simulink model "integrator_12B"  (R2022b)
settings: Solver=VariableStepAuto  StartTime=0.0  StopTime=20  RelTol=1e-3
values from neighbouring files (symbols this model uses):
  BL = -10    [SettingTUI.m]
  TL = 10    [SettingTUI.m]
undefined symbols (not defined in the file or in its folder): Hecate_Amp, Hecate_Freq
libraries: simulink x1
settings Model: LastModifiedBy=fedformi_new
settings DataIOCC: SaveFormat=Array  TimeSaveName=tOut  OutputSaveName=yOut
settings OptimizationCC: BlockReduction=off  BooleanDataType=off
settings DebuggingCC: SaveWithParameterizedLinksMsg=none  UnderspecifiedInitializationDetection=Classic  MergeDetectMultiDrivingBlocksExec=none  SignalResolutionControl=TryResolveAllWithWarning
settings HardwareCC: TargetUnknown=on
settings ModelReferenceCC: EnableRefExpFcnMdlSchedulingChecks=on  PropagateSignalLabelsOutOfModel=off

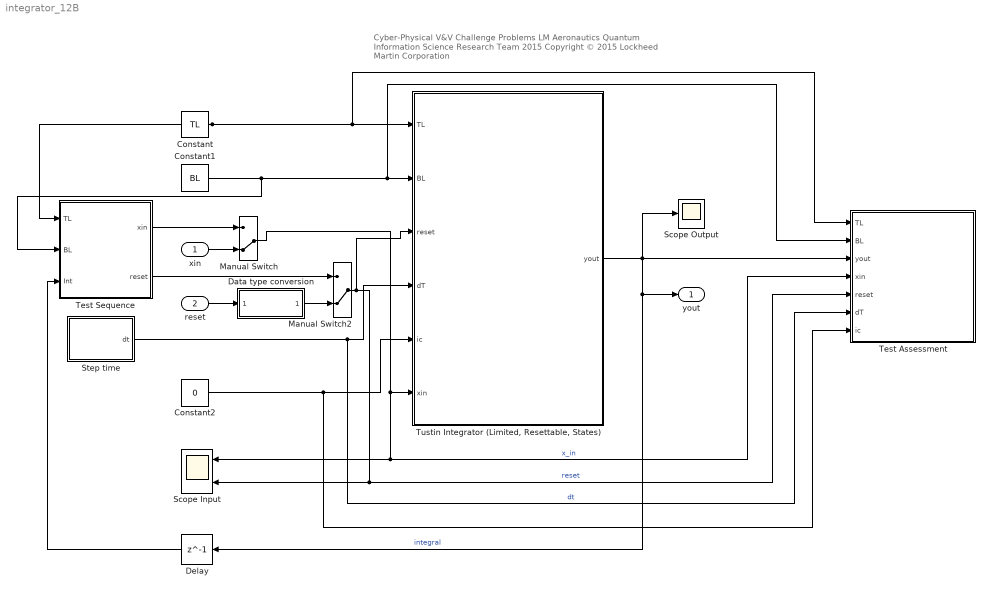
== system integrator_12B ==
  note: Cyber-Physical V&V Challenge Problems
      | LM Aeronautics Quantum Information Science Research Team 2015
      | Copyright © 2015 Lockheed Martin Corporation
  xin : Inport  OutDataTypeStr=double
  reset : Inport  Port=2
  Constant : Constant  Value=TL
  Constant1 : Constant  Value=BL
  Constant2 : Constant  Value=0
  Data type conversion : Subsystem
  Delay : Delay  DelayLength=1  InitialCondition=0
  Manual Switch : ManualSwitch  CurrentSetting=0
  Manual Switch2 : ManualSwitch  CurrentSetting=0
  Scope Input : Scope  NumInputPorts=2
  Scope Output : Scope
  Step time : Subsystem
  Test Assessment : Test Sequence  TreatAsAtomicUnit=on
  Test Sequence : Test Sequence  TreatAsAtomicUnit=on
  "Tustin Integrator (Limited, Resettable, States)" : Subsystem
  yout : Outport
  wires:
  "Tustin Integrator (Limited, Resettable, States)"/1(yout) -> Delay/1, yout/1, Scope Output/1, Test Assessment/3(yout)  "integral"
  Manual Switch/1 -> "Tustin Integrator (Limited, Resettable, States)"/6(xin), Scope Input/1, Test Assessment/4(xin)  "x_in"
  Test Sequence/1(xin) -> Manual Switch/1
  xin/1 -> Manual Switch/2
  Test Sequence/2(reset) -> Manual Switch2/1
  Constant/1 -> "Tustin Integrator (Limited, Resettable, States)"/1(TL), Test Assessment/1(TL), Test Sequence/1(TL)
  Constant1/1 -> Test Sequence/2(BL), "Tustin Integrator (Limited, Resettable, States)"/2(BL), Test Assessment/2(BL)
  Step time/1(dt) -> "Tustin Integrator (Limited, Resettable, States)"/4(dT), Test Assessment/6(dT)  "dt"
  Constant2/1 -> Test Assessment/7(ic), "Tustin Integrator (Limited, Resettable, States)"/5(ic)
  Manual Switch2/1 -> Test Assessment/5(reset), Scope Input/2, "Tustin Integrator (Limited, Resettable, States)"/3(reset)  "reset"
  reset/1 -> Data type conversion/1(reset_double)
  Data type conversion/1(reset_bool) -> Manual Switch2/2
  Delay/1 -> Test Sequence/3(Int)

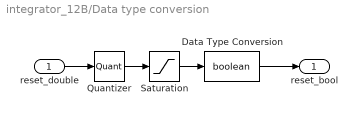
== system integrator_12B/Data type conversion ==
  reset_double : Inport  OutDataTypeStr=double
  Data Type Conversion : DataTypeConversion  OutDataTypeStr=boolean  SaturateOnIntegerOverflow=off  RndMeth=Floor
  Quantizer : Quantizer  QuantizationInterval=1
  Saturation : Saturate  UpperLimit=1  LowerLimit=0
  reset_bool : Outport
  wires:
  reset_double/1 -> Quantizer/1
  Quantizer/1 -> Saturation/1
  Data Type Conversion/1 -> reset_bool/1
  Saturation/1 -> Data Type Conversion/1

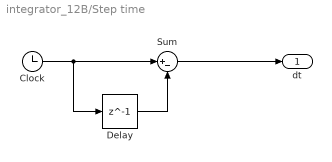
== system integrator_12B/Step time ==
  Clock : Clock
  Delay : Delay  DelayLength=1  InitialCondition=0
  Sum : Sum  Inputs=|+-
  dt : Outport
  wires:
  Sum/1 -> dt/1
  Delay/1 -> Sum/2
  Clock/1 -> Sum/1, Delay/1

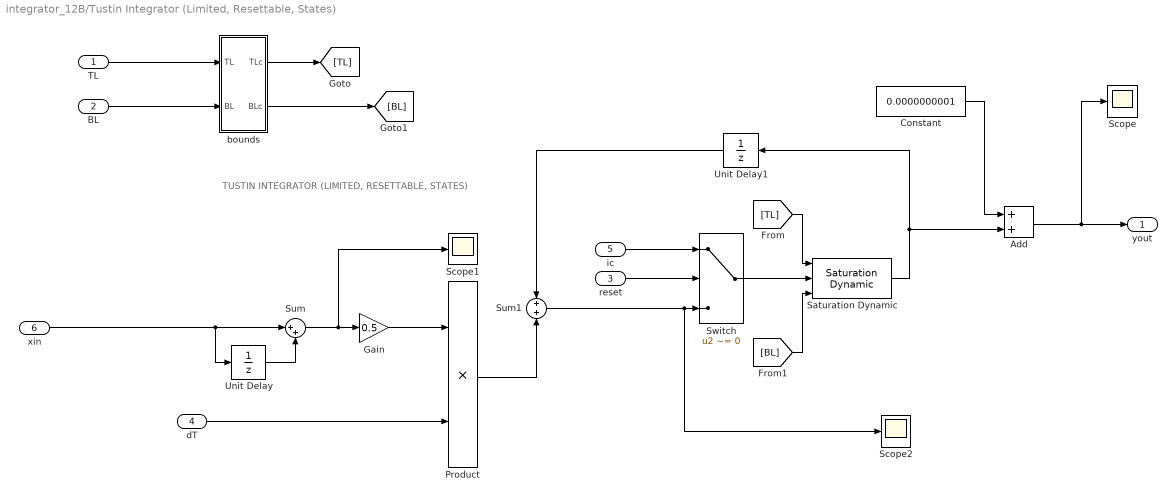
== system integrator_12B/Tustin Integrator (Limited, Resettable, States) ==
  note: TUSTIN INTEGRATOR (LIMITED, RESETTABLE, STATES)
  TL : Inport
  BL : Inport  Port=2
  reset : Inport  Port=3
  dT : Inport  Port=4
  ic : Inport  Port=5
  xin : Inport  Port=6
  Add : Sum
  Constant : Constant  Value=0.0000000001
  Gain : Gain  Gain=0.5
  Product : Product  RndMeth=Zero
  Saturation Dynamic : simulink/Discontinuities/Saturation Dynamic  OutMin=[]  OutMax=[]  OutDataTypeStr=Inherit: Same as second input  OutDataType=fixdt(1, 16)  OutScaling=2^-10  DoSatur=off
  Scope : Scope
  Scope1 : Scope
  Scope2 : Scope
  Sum : Sum  Inputs=|++
  Sum1 : Sum
  Switch : Switch  Criteria=u2 ~= 0  Threshold=0.5  SaturateOnIntegerOverflow=off  InputSameDT=off
  Unit Delay : UnitDelay  SampleTime=-1  HasFrameUpgradeWarning=on
  Unit Delay1 : UnitDelay  SampleTime=-1  HasFrameUpgradeWarning=on
  bounds : Subsystem
  yout : Outport
  wires:
  Unit Delay/1 -> Sum/2
  Sum/1 -> Scope1/1, Gain/1
  Gain/1 -> Product/1
  dT/1 -> Product/2
  Product/1 -> Sum1/2
  ic/1 -> Switch/1
  Switch/1 -> Saturation Dynamic/2
  Unit Delay1/1 -> Sum1/1
  TL/1 -> bounds/1(TL)
  BL/1 -> bounds/2(BL)
  bounds/1(TLc) -> [TL]
  bounds/2(BLc) -> [BL]
  [TL] -> Saturation Dynamic/1
  [BL] -> Saturation Dynamic/3
  Add/1 -> Scope/1, yout/1
  xin/1 -> Unit Delay/1, Sum/1
  reset/1 -> Switch/2
  Sum1/1 -> Scope2/1, Switch/3
  Saturation Dynamic/1 -> Add/2, Unit Delay1/1
  Constant/1 -> Add/1

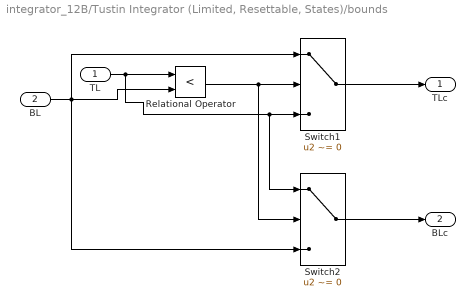
== system integrator_12B/Tustin Integrator (Limited, Resettable, States)/bounds ==
  TL : Inport
  BL : Inport  Port=2
  Relational Operator : RelationalOperator  Operator=<  OutDataTypeStr=boolean  InputSameDT=off
  Switch1 : Switch  Criteria=u2 ~= 0  Threshold=0.5  SaturateOnIntegerOverflow=off  InputSameDT=off
  Switch2 : Switch  Criteria=u2 ~= 0  Threshold=0.5  SaturateOnIntegerOverflow=off  InputSameDT=off
  TLc : Outport
  BLc : Outport  Port=2
  wires:
  BL/1 -> Switch1/1, Switch2/3, Relational Operator/2
  TL/1 -> Switch2/1, Switch1/3, Relational Operator/1
  Relational Operator/1 -> Switch2/2, Switch1/2
  Switch1/1 -> TLc/1
  Switch2/1 -> BLc/1

== stateflow chart integrator_12B/Test Assessment ==
  state step_1
    %verify(yout>=sin(t)-0.1 && yout<=sin(t)+0.1);
    %verify(yout<=10.01 && yout >=9.99);
    verify(yout <= TL && yout >= BL)
  (default) -> step_1
  data: TL input; BL input; yout input; xin input; reset input; dT input; ic input

== stateflow chart integrator_12B/Test Sequence ==
  state TUI2
    state step_1
      reset = false;
      xin=0.5+Hecate_Amp;
    state step_2
      xin=0.5+Hecate_Freq;
    (default) -> step_1
    step_1 -> step_2 : [
        | after(10,sec)
        | ]
  (default) -> TUI2 : {assert(Active_Scenario_Index == 1,'The value of Scenario Parameter ''Active_Scenario_Index'' is not valid. Use the index of the scenario to specify it.')}
  data: xin output; reset output; TL input; BL input; Hecate_Amp parameter; Hecate_Freq parameter; Int input; Active_Scenario_Index parameter =1
